simulink model "test_mdl1"  (R2023a)
settings: Solver=VariableStepAuto  StartTime=0.0  StopTime=10.0  RelTol=1e-3
(part 5 of 8)

== system test_mdl1/VehicleCAN/GWM/Power_Liftgate_Stat_FD1 ==
  DrLckCnt_No_ActlTgate : Constant  Value=0
  DrTGate_D_Rq : Constant  Value=0
  DrTgateChime2_D_Rq : Constant  Value=0
  Power_Liftgate_Mode_Stt : Constant  Value=0
  PwLftgtIntSw_B_Stat : Constant  Value=0
  bus_creator : BusCreator  Inputs=5
  out_port : Outport
  wires:
  bus_creator/1 -> out_port/1  "test_mdl1"
  DrLckCnt_No_ActlTgate/1 -> bus_creator/1  "DrLckCnt_No_ActlTgate"
  DrTGate_D_Rq/1 -> bus_creator/2  "DrTGate_D_Rq"
  DrTgateChime2_D_Rq/1 -> bus_creator/3  "DrTgateChime2_D_Rq"
  Power_Liftgate_Mode_Stt/1 -> bus_creator/4  "Power_Liftgate_Mode_Stt"
  PwLftgtIntSw_B_Stat/1 -> bus_creator/5  "PwLftgtIntSw_B_Stat"

== system test_mdl1/VehicleCAN/GWM/RCMSerialNumber_FD1 ==
  RCMSerialNoByte{1..8} (8 alike) : Constant  Value=0
  bus_creator : BusCreator  Inputs=8
  out_port : Outport
  wires:
  bus_creator/1 -> out_port/1  "test_mdl1"
  RCMSerialNoByte1/1 -> bus_creator/1  "RCMSerialNoByte1"
  RCMSerialNoByte2/1 -> bus_creator/2  "RCMSerialNoByte2"
  RCMSerialNoByte3/1 -> bus_creator/3  "RCMSerialNoByte3"
  RCMSerialNoByte4/1 -> bus_creator/4  "RCMSerialNoByte4"
  RCMSerialNoByte5/1 -> bus_creator/5  "RCMSerialNoByte5"
  RCMSerialNoByte6/1 -> bus_creator/6  "RCMSerialNoByte6"
  RCMSerialNoByte7/1 -> bus_creator/7  "RCMSerialNoByte7"
  RCMSerialNoByte8/1 -> bus_creator/8  "RCMSerialNoByte8"

== system test_mdl1/VehicleCAN/GWM/RCMStatusMessage2_FD1 ==
  EDRTriggerEvntSync : Constant  Value=0
  FirstRowBuckleDriver : Constant  Value=0
  FirstRowBuckleMid : Constant  Value=0
  FirstRowBucklePsngr : Constant  Value=0
  PassRstrnInd_Req : Constant  Value=0
  PsngrFrntDetct_D_Actl : Constant  Value=0
  RILReq : Constant  Value=0
  RstrnImpactEvntStatus : Constant  Value=0
  SecondRowBuckleDriver : Constant  Value=0
  SecondRowBuckleMid : Constant  Value=0
  SecondRowBucklePsngr : Constant  Value=0
  bus_creator : BusCreator  Inputs=11
  out_port : Outport
  wires:
  bus_creator/1 -> out_port/1  "test_mdl1"
  EDRTriggerEvntSync/1 -> bus_creator/1  "EDRTriggerEvntSync"
  FirstRowBuckleDriver/1 -> bus_creator/2  "FirstRowBuckleDriver"
  FirstRowBuckleMid/1 -> bus_creator/3  "FirstRowBuckleMid"
  FirstRowBucklePsngr/1 -> bus_creator/4  "FirstRowBucklePsngr"
  PassRstrnInd_Req/1 -> bus_creator/5  "PassRstrnInd_Req"
  PsngrFrntDetct_D_Actl/1 -> bus_creator/6  "PsngrFrntDetct_D_Actl"
  RILReq/1 -> bus_creator/7  "RILReq"
  RstrnImpactEvntStatus/1 -> bus_creator/8  "RstrnImpactEvntStatus"
  SecondRowBuckleDriver/1 -> bus_creator/9  "SecondRowBuckleDriver"
  SecondRowBuckleMid/1 -> bus_creator/10  "SecondRowBuckleMid"
  SecondRowBucklePsngr/1 -> bus_creator/11  "SecondRowBucklePsngr"

== system test_mdl1/VehicleCAN/GWM/SmartChargingData_ECG_1 ==
  ScLocDelete_B_RqCld : Constant  Value=0
  ScLocId_No_RqCld : Constant  Value=0
  ScLocLattDeg_An_RqCld : Constant  Value=0
  ScLocLattFrct_An_RqCld : Constant  Value=0
  ScLocLattPostv_B_RqCld : Constant  Value=0
  ScLocLongDeg_An_RqCld : Constant  Value=0
  ScLocLongFrct_An_RqCld : Constant  Value=0
  ScLocLongPostv_B_RqCld : Constant  Value=0
  bus_creator : BusCreator  Inputs=8
  out_port : Outport
  wires:
  bus_creator/1 -> out_port/1  "test_mdl1"
  ScLocDelete_B_RqCld/1 -> bus_creator/1  "ScLocDelete_B_RqCld"
  ScLocId_No_RqCld/1 -> bus_creator/2  "ScLocId_No_RqCld"
  ScLocLattDeg_An_RqCld/1 -> bus_creator/3  "ScLocLattDeg_An_RqCld"
  ScLocLattFrct_An_RqCld/1 -> bus_creator/4  "ScLocLattFrct_An_RqCld"
  ScLocLattPostv_B_RqCld/1 -> bus_creator/5  "ScLocLattPostv_B_RqCld"
  ScLocLongDeg_An_RqCld/1 -> bus_creator/6  "ScLocLongDeg_An_RqCld"
  ScLocLongFrct_An_RqCld/1 -> bus_creator/7  "ScLocLongFrct_An_RqCld"
  ScLocLongPostv_B_RqCld/1 -> bus_creator/8  "ScLocLongPostv_B_RqCld"

== system test_mdl1/VehicleCAN/GWM/SmartChargingData_ECG_2 ==
  ScChrgDurSet_D_RqCld : Constant  Value=0
  ScChrgDur_T_RqCld : Constant  Value=0
  ScChrgPrfl_No_RqCld : Constant  Value=0
  ScChrgToPc_Pc_RqCld : Constant  Value=0
  ScDayOfWeekId_D_RqCld : Constant  Value=0
  ScLocRdius_L_RqCld : Constant  Value=0
  ScLocSetId_No_RqCld : Constant  Value=0
  bus_creator : BusCreator  Inputs=7
  out_port : Outport
  wires:
  bus_creator/1 -> out_port/1  "test_mdl1"
  ScChrgDurSet_D_RqCld/1 -> bus_creator/1  "ScChrgDurSet_D_RqCld"
  ScChrgDur_T_RqCld/1 -> bus_creator/2  "ScChrgDur_T_RqCld"
  ScChrgPrfl_No_RqCld/1 -> bus_creator/3  "ScChrgPrfl_No_RqCld"
  ScChrgToPc_Pc_RqCld/1 -> bus_creator/4  "ScChrgToPc_Pc_RqCld"
  ScDayOfWeekId_D_RqCld/1 -> bus_creator/5  "ScDayOfWeekId_D_RqCld"
  ScLocRdius_L_RqCld/1 -> bus_creator/6  "ScLocRdius_L_RqCld"
  ScLocSetId_No_RqCld/1 -> bus_creator/7  "ScLocSetId_No_RqCld"

== system test_mdl1/VehicleCAN/GWM/SmartChargingData_ECG_3 ==
  AirAmb_Te_ActlCld : Constant  Value=0
  ChrgToPcEdit_Pc_RqCld : Constant  Value=0
  GoTEditHr_T_RqCld : Constant  Value=0
  GoTEditMnte_T_RqCld : Constant  Value=0
  PrcondEdit_D_RqCld : Constant  Value=0
  ScChrgrPwMax_Pw_RqCld : Constant  Value=0
  ScEnbl_D_RqCld : Constant  Value=0
  ScFreshDataEnbl_B_Rq : Constant  Value=0
  ScLocPwId_No_RqCld : Constant  Value=0
  ScMnSoc_Pc_RqCld : Constant  Value=0
  bus_creator : BusCreator  Inputs=10
  out_port : Outport
  wires:
  bus_creator/1 -> out_port/1  "test_mdl1"
  AirAmb_Te_ActlCld/1 -> bus_creator/1  "AirAmb_Te_ActlCld"
  ChrgToPcEdit_Pc_RqCld/1 -> bus_creator/2  "ChrgToPcEdit_Pc_RqCld"
  GoTEditHr_T_RqCld/1 -> bus_creator/3  "GoTEditHr_T_RqCld"
  GoTEditMnte_T_RqCld/1 -> bus_creator/4  "GoTEditMnte_T_RqCld"
  PrcondEdit_D_RqCld/1 -> bus_creator/5  "PrcondEdit_D_RqCld"
  ScChrgrPwMax_Pw_RqCld/1 -> bus_creator/6  "ScChrgrPwMax_Pw_RqCld"
  ScEnbl_D_RqCld/1 -> bus_creator/7  "ScEnbl_D_RqCld"
  ScFreshDataEnbl_B_Rq/1 -> bus_creator/8  "ScFreshDataEnbl_B_Rq"
  ScLocPwId_No_RqCld/1 -> bus_creator/9  "ScLocPwId_No_RqCld"
  ScMnSoc_Pc_RqCld/1 -> bus_creator/10  "ScMnSoc_Pc_RqCld"

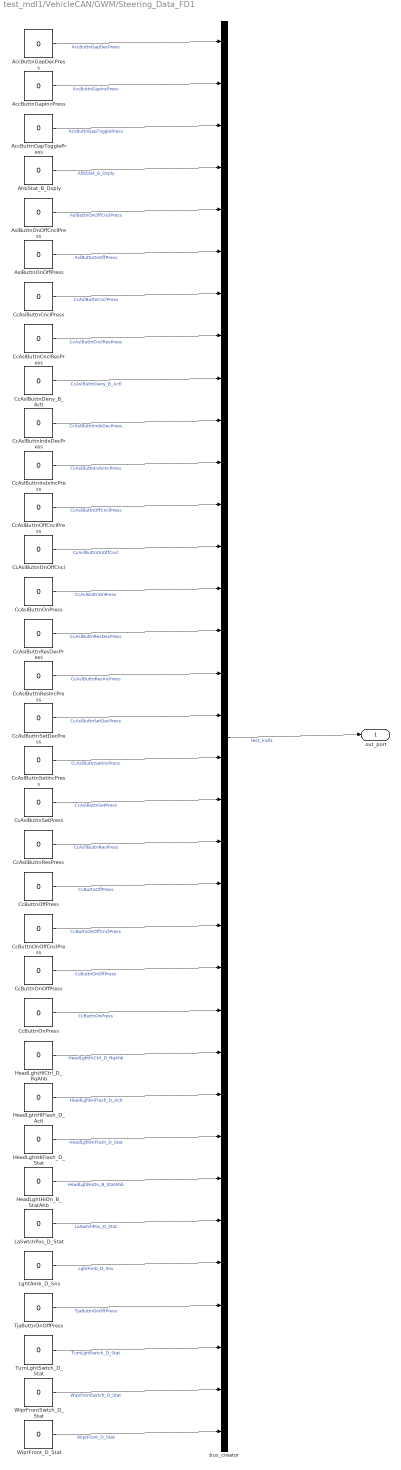
== system test_mdl1/VehicleCAN/GWM/Steering_Data_FD1 ==
  AccButtnGapDecPress : Constant  Value=0
  AccButtnGapIncPress : Constant  Value=0
  AccButtnGapTogglePress : Constant  Value=0
  AhbStat_B_Dsply : Constant  Value=0
  AslButtnOnOffCnclPress : Constant  Value=0
  AslButtnOnOffPress : Constant  Value=0
  CcAslButtnCnclPress : Constant  Value=0
  CcAslButtnCnclResPress : Constant  Value=0
  CcAslButtnDeny_B_Actl : Constant  Value=0
  CcAslButtnIndxDecPress : Constant  Value=0
  CcAslButtnIndxIncPress : Constant  Value=0
  CcAslButtnOffCnclPress : Constant  Value=0
  CcAslButtnOnOffCncl : Constant  Value=0
  CcAslButtnOnPress : Constant  Value=0
  CcAslButtnResDecPress : Constant  Value=0
  CcAslButtnResIncPress : Constant  Value=0
  CcAslButtnSetDecPress : Constant  Value=0
  CcAslButtnSetIncPress : Constant  Value=0
  CcAslButtnSetPress : Constant  Value=0
  CcAsllButtnResPress : Constant  Value=0
  CcButtnOffPress : Constant  Value=0
  CcButtnOnOffCnclPress : Constant  Value=0
  CcButtnOnOffPress : Constant  Value=0
  CcButtnOnPress : Constant  Value=0
  HeadLghtHiCtrl_D_RqAhb : Constant  Value=0
  HeadLghtHiFlash_D_Actl : Constant  Value=0
  HeadLghtHiFlash_D_Stat : Constant  Value=0
  HeadLghtHiOn_B_StatAhb : Constant  Value=0
  LaSwtchPos_D_Stat : Constant  Value=0
  LghtAmb_D_Sns : Constant  Value=0
  TjaButtnOnOffPress : Constant  Value=0
  TurnLghtSwtch_D_Stat : Constant  Value=0
  WiprFrontSwtch_D_Stat : Constant  Value=0
  WiprFront_D_Stat : Constant  Value=0
  bus_creator : BusCreator  Inputs=34
  out_port : Outport
  wires:
  bus_creator/1 -> out_port/1  "test_mdl1"
  AccButtnGapDecPress/1 -> bus_creator/1  "AccButtnGapDecPress"
  AccButtnGapIncPress/1 -> bus_creator/2  "AccButtnGapIncPress"
  AccButtnGapTogglePress/1 -> bus_creator/3  "AccButtnGapTogglePress"
  AhbStat_B_Dsply/1 -> bus_creator/4  "AhbStat_B_Dsply"
  AslButtnOnOffCnclPress/1 -> bus_creator/5  "AslButtnOnOffCnclPress"
  AslButtnOnOffPress/1 -> bus_creator/6  "AslButtnOnOffPress"
  CcAslButtnCnclPress/1 -> bus_creator/7  "CcAslButtnCnclPress"
  CcAslButtnCnclResPress/1 -> bus_creator/8  "CcAslButtnCnclResPress"
  CcAslButtnDeny_B_Actl/1 -> bus_creator/9  "CcAslButtnDeny_B_Actl"
  CcAslButtnIndxDecPress/1 -> bus_creator/10  "CcAslButtnIndxDecPress"
  CcAslButtnIndxIncPress/1 -> bus_creator/11  "CcAslButtnIndxIncPress"
  CcAslButtnOffCnclPress/1 -> bus_creator/12  "CcAslButtnOffCnclPress"
  CcAslButtnOnOffCncl/1 -> bus_creator/13  "CcAslButtnOnOffCncl"
  CcAslButtnOnPress/1 -> bus_creator/14  "CcAslButtnOnPress"
  CcAslButtnResDecPress/1 -> bus_creator/15  "CcAslButtnResDecPress"
  CcAslButtnResIncPress/1 -> bus_creator/16  "CcAslButtnResIncPress"
  CcAslButtnSetDecPress/1 -> bus_creator/17  "CcAslButtnSetDecPress"
  CcAslButtnSetIncPress/1 -> bus_creator/18  "CcAslButtnSetIncPress"
  CcAslButtnSetPress/1 -> bus_creator/19  "CcAslButtnSetPress"
  CcAsllButtnResPress/1 -> bus_creator/20  "CcAsllButtnResPress"
  CcButtnOffPress/1 -> bus_creator/21  "CcButtnOffPress"
  CcButtnOnOffCnclPress/1 -> bus_creator/22  "CcButtnOnOffCnclPress"
  CcButtnOnOffPress/1 -> bus_creator/23  "CcButtnOnOffPress"
  CcButtnOnPress/1 -> bus_creator/24  "CcButtnOnPress"
  HeadLghtHiCtrl_D_RqAhb/1 -> bus_creator/25  "HeadLghtHiCtrl_D_RqAhb"
  HeadLghtHiFlash_D_Actl/1 -> bus_creator/26  "HeadLghtHiFlash_D_Actl"
  HeadLghtHiFlash_D_Stat/1 -> bus_creator/27  "HeadLghtHiFlash_D_Stat"
  HeadLghtHiOn_B_StatAhb/1 -> bus_creator/28  "HeadLghtHiOn_B_StatAhb"
  LaSwtchPos_D_Stat/1 -> bus_creator/29  "LaSwtchPos_D_Stat"
  LghtAmb_D_Sns/1 -> bus_creator/30  "LghtAmb_D_Sns"
  TjaButtnOnOffPress/1 -> bus_creator/31  "TjaButtnOnOffPress"
  TurnLghtSwtch_D_Stat/1 -> bus_creator/32  "TurnLghtSwtch_D_Stat"
  WiprFrontSwtch_D_Stat/1 -> bus_creator/33  "WiprFrontSwtch_D_Stat"
  WiprFront_D_Stat/1 -> bus_creator/34  "WiprFront_D_Stat"

== system test_mdl1/VehicleCAN/GWM/Steering_Wheel_Data2_FD1 ==
  SelDrvMdeDec_B_RqDrv : Constant  Value=0
  SelDrvMdeInc_B_RqDrv : Constant  Value=0
  SelDrvMdeSwtch_D_Stat4 : Constant  Value=0
  SteEffortInc_B_RqDrv : Constant  Value=0
  SteWhlSwtchBack_B_Stat : Constant  Value=0
  SteWhlSwtchDown_B_Stat : Constant  Value=0
  SteWhlSwtchHome_B_Stat : Constant  Value=0
  SteWhlSwtchHud_B_Stat : Constant  Value=0
  SteWhlSwtchInfo_B_Stat : Constant  Value=0
  SteWhlSwtchIod_B_Stat : Constant  Value=0
  SteWhlSwtchLeft_B_Stat : Constant  Value=0
  SteWhlSwtchMed_B_Stat : Constant  Value=0
  SteWhlSwtchMenu_B_Stat : Constant  Value=0
  SteWhlSwtchNav_B_Stat : Constant  Value=0
  SteWhlSwtchOk_B_Stat : Constant  Value=0
  SteWhlSwtchPhon_B_Stat : Constant  Value=0
  SteWhlSwtchRght_B_Stat : Constant  Value=0
  SteWhlSwtchSet_B_Stat : Constant  Value=0
  SteWhlSwtchUp_B_Stat : Constant  Value=0
  SteWhlSwtchView_B_Stat : Constant  Value=0
  SuspDampInc_B_RqDrv : Constant  Value=0
  bus_creator : BusCreator  Inputs=21
  out_port : Outport
  wires:
  bus_creator/1 -> out_port/1  "test_mdl1"
  SelDrvMdeDec_B_RqDrv/1 -> bus_creator/1  "SelDrvMdeDec_B_RqDrv"
  SelDrvMdeInc_B_RqDrv/1 -> bus_creator/2  "SelDrvMdeInc_B_RqDrv"
  SelDrvMdeSwtch_D_Stat4/1 -> bus_creator/3  "SelDrvMdeSwtch_D_Stat4"
  SteEffortInc_B_RqDrv/1 -> bus_creator/4  "SteEffortInc_B_RqDrv"
  SteWhlSwtchBack_B_Stat/1 -> bus_creator/5  "SteWhlSwtchBack_B_Stat"
  SteWhlSwtchDown_B_Stat/1 -> bus_creator/6  "SteWhlSwtchDown_B_Stat"
  SteWhlSwtchHome_B_Stat/1 -> bus_creator/7  "SteWhlSwtchHome_B_Stat"
  SteWhlSwtchHud_B_Stat/1 -> bus_creator/8  "SteWhlSwtchHud_B_Stat"
  SteWhlSwtchInfo_B_Stat/1 -> bus_creator/9  "SteWhlSwtchInfo_B_Stat"
  SteWhlSwtchIod_B_Stat/1 -> bus_creator/10  "SteWhlSwtchIod_B_Stat"
  SteWhlSwtchLeft_B_Stat/1 -> bus_creator/11  "SteWhlSwtchLeft_B_Stat"
  SteWhlSwtchMed_B_Stat/1 -> bus_creator/12  "SteWhlSwtchMed_B_Stat"
  SteWhlSwtchMenu_B_Stat/1 -> bus_creator/13  "SteWhlSwtchMenu_B_Stat"
  SteWhlSwtchNav_B_Stat/1 -> bus_creator/14  "SteWhlSwtchNav_B_Stat"
  SteWhlSwtchOk_B_Stat/1 -> bus_creator/15  "SteWhlSwtchOk_B_Stat"
  SteWhlSwtchPhon_B_Stat/1 -> bus_creator/16  "SteWhlSwtchPhon_B_Stat"
  SteWhlSwtchRght_B_Stat/1 -> bus_creator/17  "SteWhlSwtchRght_B_Stat"
  SteWhlSwtchSet_B_Stat/1 -> bus_creator/18  "SteWhlSwtchSet_B_Stat"
  SteWhlSwtchUp_B_Stat/1 -> bus_creator/19  "SteWhlSwtchUp_B_Stat"
  SteWhlSwtchView_B_Stat/1 -> bus_creator/20  "SteWhlSwtchView_B_Stat"
  SuspDampInc_B_RqDrv/1 -> bus_creator/21  "SuspDampInc_B_RqDrv"

== system test_mdl1/VehicleCAN/GWM/TCU_Send_Signals_FD1 ==
  EmgcyCallMute_D_Stat : Constant  Value=0
  OfbChrgSetSync_D_Rq : Constant  Value=0
  TelematicsSrvc_D_St : Constant  Value=0
  bus_creator : BusCreator  Inputs=3
  out_port : Outport
  wires:
  bus_creator/1 -> out_port/1  "test_mdl1"
  EmgcyCallMute_D_Stat/1 -> bus_creator/1  "EmgcyCallMute_D_Stat"
  OfbChrgSetSync_D_Rq/1 -> bus_creator/2  "OfbChrgSetSync_D_Rq"
  TelematicsSrvc_D_St/1 -> bus_creator/3  "TelematicsSrvc_D_St"

== system test_mdl1/VehicleCAN/GWM/TesterPhysicalReqVDM_FD1 ==
  TesterPhysicalReqVDM : Constant  Value=0
  bus_creator : BusCreator  Inputs=1
  out_port : Outport
  wires:
  bus_creator/1 -> out_port/1  "test_mdl1"
  TesterPhysicalReqVDM/1 -> bus_creator/1  "TesterPhysicalReqVDM"

== system test_mdl1/VehicleCAN/GWM/TesterPhysicalResGWM_FD1 ==
  TesterPhysicalResGWM_F1 : Constant  Value=0
  bus_creator : BusCreator  Inputs=1
  out_port : Outport
  wires:
  bus_creator/1 -> out_port/1  "test_mdl1"
  TesterPhysicalResGWM_F1/1 -> bus_creator/1  "TesterPhysicalResGWM_F1"

== system test_mdl1/VehicleCAN/GWM/Tire_Pressure_Data_FD1 ==
  Tire_Press_LF_Data : Constant  Value=0
  Tire_Press_LR_OLR_Data : Constant  Value=0
  Tire_Press_RF_Data : Constant  Value=0
  Tire_Press_RR_ORR_Data : Constant  Value=0
  bus_creator : BusCreator  Inputs=4
  out_port : Outport
  wires:
  bus_creator/1 -> out_port/1  "test_mdl1"
  Tire_Press_LF_Data/1 -> bus_creator/1  "Tire_Press_LF_Data"
  Tire_Press_LR_OLR_Data/1 -> bus_creator/2  "Tire_Press_LR_OLR_Data"
  Tire_Press_RF_Data/1 -> bus_creator/3  "Tire_Press_RF_Data"
  Tire_Press_RR_ORR_Data/1 -> bus_creator/4  "Tire_Press_RR_ORR_Data"

== system test_mdl1/VehicleCAN/GWM/TrailerAid_Data3_FD1 ==
  TrlrAidEnbl_D2_Rq : Constant  Value=0
  TrlrAidSetup_D2_Rq : Constant  Value=0
  TrlrAnOffstDir_D_Mem : Constant  Value=0
  TrlrAnOffst_An_Mem : Constant  Value=0
  TrlrAxleToBmpr_L_Actl : Constant  Value=0
  TrlrBallToBmpr_L_Actl : Constant  Value=0
  TrlrIdType_D_Stat : Constant  Value=0
  TrlrId_No_Actl : Constant  Value=0
  TrlrRvrseCancl_B_Rq : Constant  Value=0
  TrlrTrgtOffst_L_Actl : Constant  Value=0
  TrlrTrgtPtrnId_No_Mem : Constant  Value=0
  TrlrTrgtToBmpr_L_Actl : Constant  Value=0
  bus_creator : BusCreator  Inputs=12
  out_port : Outport
  wires:
  bus_creator/1 -> out_port/1  "test_mdl1"
  TrlrAidEnbl_D2_Rq/1 -> bus_creator/1  "TrlrAidEnbl_D2_Rq"
  TrlrAidSetup_D2_Rq/1 -> bus_creator/2  "TrlrAidSetup_D2_Rq"
  TrlrAnOffstDir_D_Mem/1 -> bus_creator/3  "TrlrAnOffstDir_D_Mem"
  TrlrAnOffst_An_Mem/1 -> bus_creator/4  "TrlrAnOffst_An_Mem"
  TrlrAxleToBmpr_L_Actl/1 -> bus_creator/5  "TrlrAxleToBmpr_L_Actl"
  TrlrBallToBmpr_L_Actl/1 -> bus_creator/6  "TrlrBallToBmpr_L_Actl"
  TrlrIdType_D_Stat/1 -> bus_creator/7  "TrlrIdType_D_Stat"
  TrlrId_No_Actl/1 -> bus_creator/8  "TrlrId_No_Actl"
  TrlrRvrseCancl_B_Rq/1 -> bus_creator/9  "TrlrRvrseCancl_B_Rq"
  TrlrTrgtOffst_L_Actl/1 -> bus_creator/10  "TrlrTrgtOffst_L_Actl"
  TrlrTrgtPtrnId_No_Mem/1 -> bus_creator/11  "TrlrTrgtPtrnId_No_Mem"
  TrlrTrgtToBmpr_L_Actl/1 -> bus_creator/12  "TrlrTrgtToBmpr_L_Actl"

== system test_mdl1/VehicleCAN/GWM/TrailerAid_Data_FD1 ==
  TrailCtlSwtch_B_Stat2 : Constant  Value=0
  TrlBrkInitOut_D_Rq : Constant  Value=0
  bus_creator : BusCreator  Inputs=2
  out_port : Outport
  wires:
  bus_creator/1 -> out_port/1  "test_mdl1"
  TrailCtlSwtch_B_Stat2/1 -> bus_creator/1  "TrailCtlSwtch_B_Stat2"
  TrlBrkInitOut_D_Rq/1 -> bus_creator/2  "TrlBrkInitOut_D_Rq"

== system test_mdl1/VehicleCAN/GWM/TrailerAid_Stat1_FD1 ==
  TrlrSnsId_No_Actl : Constant  Value=0
  bus_creator : BusCreator  Inputs=1
  out_port : Outport
  wires:
  bus_creator/1 -> out_port/1  "test_mdl1"
  TrlrSnsId_No_Actl/1 -> bus_creator/1  "TrlrSnsId_No_Actl"

== system test_mdl1/VehicleCAN/GWM/TrailerAid_Stat2_FD1 ==
  TrlrHitYaw_AnRate_Actl : Constant  Value=0
  TrlrHitchYaw_An_Actl : Constant  Value=0
  TrlrHitchYaw_D_Stat : Constant  Value=0
  TrlrYawWActl_D_Qf : Constant  Value=0
  TrlrYaw_W_Actl : Constant  Value=0
  bus_creator : BusCreator  Inputs=5
  out_port : Outport
  wires:
  bus_creator/1 -> out_port/1  "test_mdl1"
  TrlrHitYaw_AnRate_Actl/1 -> bus_creator/1  "TrlrHitYaw_AnRate_Actl"
  TrlrHitchYaw_An_Actl/1 -> bus_creator/2  "TrlrHitchYaw_An_Actl"
  TrlrHitchYaw_D_Stat/1 -> bus_creator/3  "TrlrHitchYaw_D_Stat"
  TrlrYawWActl_D_Qf/1 -> bus_creator/4  "TrlrYawWActl_D_Qf"
  TrlrYaw_W_Actl/1 -> bus_creator/5  "TrlrYaw_W_Actl"

== system test_mdl1/VehicleCAN/GWM/TrailerBrakeInfo_FD1 ==
  StopLamp_B_RqTrlrBrk : Constant  Value=0
  TrlBrkInitOut_D_Stat : Constant  Value=0
  TrlrBrkActCirct_B_Falt : Constant  Value=0
  TrlrBrkActCnnct_B_Actl : Constant  Value=0
  TrlrBrkCtl_B_Falt : Constant  Value=0
  TrlrBrkDcnnt_B_Actl : Constant  Value=0
  TrlrBrkDsply_B_Rq : Constant  Value=0
  TrlrBrkGain_No_Actl : Constant  Value=0
  TrlrBrkMde_D_Actl : Constant  Value=0
  TrlrBrkOut_No_Dsply : Constant  Value=0
  bus_creator : BusCreator  Inputs=10
  out_port : Outport
  wires:
  bus_creator/1 -> out_port/1  "test_mdl1"
  StopLamp_B_RqTrlrBrk/1 -> bus_creator/1  "StopLamp_B_RqTrlrBrk"
  TrlBrkInitOut_D_Stat/1 -> bus_creator/2  "TrlBrkInitOut_D_Stat"
  TrlrBrkActCirct_B_Falt/1 -> bus_creator/3  "TrlrBrkActCirct_B_Falt"
  TrlrBrkActCnnct_B_Actl/1 -> bus_creator/4  "TrlrBrkActCnnct_B_Actl"
  TrlrBrkCtl_B_Falt/1 -> bus_creator/5  "TrlrBrkCtl_B_Falt"
  TrlrBrkDcnnt_B_Actl/1 -> bus_creator/6  "TrlrBrkDcnnt_B_Actl"
  TrlrBrkDsply_B_Rq/1 -> bus_creator/7  "TrlrBrkDsply_B_Rq"
  TrlrBrkGain_No_Actl/1 -> bus_creator/8  "TrlrBrkGain_No_Actl"
  TrlrBrkMde_D_Actl/1 -> bus_creator/9  "TrlrBrkMde_D_Actl"
  TrlrBrkOut_No_Dsply/1 -> bus_creator/10  "TrlrBrkOut_No_Dsply"

== system test_mdl1/VehicleCAN/GWM/TrailerInfo_2_FD1 ==
  TrlrAidCtl_U_RqDrv : Constant  Value=0
  TrlrAidSwtch_D_RqDrv : Constant  Value=0
  bus_creator : BusCreator  Inputs=2
  out_port : Outport
  wires:
  bus_creator/1 -> out_port/1  "test_mdl1"
  TrlrAidCtl_U_RqDrv/1 -> bus_creator/1  "TrlrAidCtl_U_RqDrv"
  TrlrAidSwtch_D_RqDrv/1 -> bus_creator/2  "TrlrAidSwtch_D_RqDrv"

== system test_mdl1/VehicleCAN/GWM/TrailerInfo_FD1 ==
  ParkLampTrlrOut_B_Stat : Constant  Value=0
  StopLampTrlrOut_B_Stat : Constant  Value=0
  TrlrBattChrg_D_Stat : Constant  Value=0
  TrlrLampCnnct_B_Actl : Constant  Value=0
  TrlrLampCtl_D_Stat : Constant  Value=0
  TurnLampTrlrRl_B_Stat : Constant  Value=0
  TurnLampTrlrRr_B_Stat : Constant  Value=0
  bus_creator : BusCreator  Inputs=7
  out_port : Outport
  wires:
  bus_creator/1 -> out_port/1  "test_mdl1"
  ParkLampTrlrOut_B_Stat/1 -> bus_creator/1  "ParkLampTrlrOut_B_Stat"
  StopLampTrlrOut_B_Stat/1 -> bus_creator/2  "StopLampTrlrOut_B_Stat"
  TrlrBattChrg_D_Stat/1 -> bus_creator/3  "TrlrBattChrg_D_Stat"
  TrlrLampCnnct_B_Actl/1 -> bus_creator/4  "TrlrLampCnnct_B_Actl"
  TrlrLampCtl_D_Stat/1 -> bus_creator/5  "TrlrLampCtl_D_Stat"
  TurnLampTrlrRl_B_Stat/1 -> bus_creator/6  "TurnLampTrlrRl_B_Stat"
  TurnLampTrlrRr_B_Stat/1 -> bus_creator/7  "TurnLampTrlrRr_B_Stat"

== system test_mdl1/VehicleCAN/GWM/Voltage_Power_Data2_FD1 ==
  CoolFanDcdc_D_Rq : Constant  Value=0
  DcdcClntFlw_D_Rq : Constant  Value=0
  bus_creator : BusCreator  Inputs=2
  out_port : Outport
  wires:
  bus_creator/1 -> out_port/1  "test_mdl1"
  CoolFanDcdc_D_Rq/1 -> bus_creator/1  "CoolFanDcdc_D_Rq"
  DcdcClntFlw_D_Rq/1 -> bus_creator/2  "DcdcClntFlw_D_Rq"

== system test_mdl1/VehicleCAN/GWM/Yaw_Data_FD1 ==
  VehRolWActl_D_Qf : Constant  Value=0
  VehRol_W_Actl : Constant  Value=0
  VehRollYawW_No_Cs : Constant  Value=0
  VehRollYaw_No_Cnt : Constant  Value=0
  VehYawWActl_D_Qf : Constant  Value=0
  VehYaw_W_Actl : Constant  Value=0
  bus_creator : BusCreator  Inputs=6
  out_port : Outport
  wires:
  bus_creator/1 -> out_port/1  "test_mdl1"
  VehRolWActl_D_Qf/1 -> bus_creator/1  "VehRolWActl_D_Qf"
  VehRol_W_Actl/1 -> bus_creator/2  "VehRol_W_Actl"
  VehRollYawW_No_Cs/1 -> bus_creator/3  "VehRollYawW_No_Cs"
  VehRollYaw_No_Cnt/1 -> bus_creator/4  "VehRollYaw_No_Cnt"
  VehYawWActl_D_Qf/1 -> bus_creator/5  "VehYawWActl_D_Qf"
  VehYaw_W_Actl/1 -> bus_creator/6  "VehYaw_W_Actl"

== system test_mdl1/VehicleCAN/IPMA_ADAS/%sonality_CCM_Data ==
  %sIndexCcm_D_Actl : Constant  Value=0
  FeatConfigCcmActl : Constant  Value=0
  FeatNoCcmActl : Constant  Value=0
  bus_creator : BusCreator  Inputs=3
  out_port : Outport
  wires:
  bus_creator/1 -> out_port/1  "test_mdl1"
  FeatConfigCcmActl/1 -> bus_creator/1  "FeatConfigCcmActl"
  FeatNoCcmActl/1 -> bus_creator/2  "FeatNoCcmActl"
  %sIndexCcm_D_Actl/1 -> bus_creator/3  "%sIndexCcm_D_Actl"

== system test_mdl1/VehicleCAN/IPMA_ADAS/%sonality_IPMB_Data ==
  %sIndexIpmb_D_Actl : Constant  Value=0
  FeatConfigIpmbActl : Constant  Value=0
  FeatNoIpmbActl : Constant  Value=0
  bus_creator : BusCreator  Inputs=3
  out_port : Outport
  wires:
  bus_creator/1 -> out_port/1  "test_mdl1"
  FeatConfigIpmbActl/1 -> bus_creator/1  "FeatConfigIpmbActl"
  FeatNoIpmbActl/1 -> bus_creator/2  "FeatNoIpmbActl"
  %sIndexIpmb_D_Actl/1 -> bus_creator/3  "%sIndexIpmb_D_Actl"

== system test_mdl1/VehicleCAN/IPMA_ADAS/ACCDATA ==
  AccAutoResum_D_Rq : Constant  Value=0
  AccBrkDecel_B_Rq : Constant  Value=0
  AccBrkPrchg_B_Rq : Constant  Value=0
  AccBrkPrkEl_B_Rq : Constant  Value=0
  AccBrkPulse_B_Rq : Constant  Value=0
  AccBrkTot_A_Rq : Constant  Value=0
  AccCancl_B_Rq : Constant  Value=0
  AccDeny_B_Rq : Constant  Value=0
  AccPrpl_A_Pred : Constant  Value=0
  AccPrpl_A_Rq : Constant  Value=0
  AccResumEnbl_B_Rq : Constant  Value=0
  AccStopStat_B_Rq : Constant  Value=0
  AccVeh_V_Trg : Constant  Value=0
  CmbbDeny_B_Actl : Constant  Value=0
  CmbbEngTqMn_B_Rq : Constant  Value=0
  CmbbOvrrd_B_RqDrv : Constant  Value=0
  Cmbb_B_Enbl : Constant  Value=0
  bus_creator : BusCreator  Inputs=17
  out_port : Outport
  wires:
  bus_creator/1 -> out_port/1  "test_mdl1"
  AccAutoResum_D_Rq/1 -> bus_creator/1  "AccAutoResum_D_Rq"
  AccBrkDecel_B_Rq/1 -> bus_creator/2  "AccBrkDecel_B_Rq"
  AccBrkPrchg_B_Rq/1 -> bus_creator/3  "AccBrkPrchg_B_Rq"
  AccBrkPrkEl_B_Rq/1 -> bus_creator/4  "AccBrkPrkEl_B_Rq"
  AccBrkPulse_B_Rq/1 -> bus_creator/5  "AccBrkPulse_B_Rq"
  AccBrkTot_A_Rq/1 -> bus_creator/6  "AccBrkTot_A_Rq"
  AccCancl_B_Rq/1 -> bus_creator/7  "AccCancl_B_Rq"
  AccDeny_B_Rq/1 -> bus_creator/8  "AccDeny_B_Rq"
  AccPrpl_A_Pred/1 -> bus_creator/9  "AccPrpl_A_Pred"
  AccPrpl_A_Rq/1 -> bus_creator/10  "AccPrpl_A_Rq"
  AccResumEnbl_B_Rq/1 -> bus_creator/11  "AccResumEnbl_B_Rq"
  AccStopStat_B_Rq/1 -> bus_creator/12  "AccStopStat_B_Rq"
  AccVeh_V_Trg/1 -> bus_creator/13  "AccVeh_V_Trg"
  CmbbDeny_B_Actl/1 -> bus_creator/14  "CmbbDeny_B_Actl"
  CmbbEngTqMn_B_Rq/1 -> bus_creator/15  "CmbbEngTqMn_B_Rq"
  CmbbOvrrd_B_RqDrv/1 -> bus_creator/16  "CmbbOvrrd_B_RqDrv"
  Cmbb_B_Enbl/1 -> bus_creator/17  "Cmbb_B_Enbl"

== system test_mdl1/VehicleCAN/IPMA_ADAS/ACCDATA_2 ==
  CmbbBaSens_D_Rq : Constant  Value=0
  CmbbBrkDecel_A_Rq : Constant  Value=0
  CmbbBrkDecel_B_Rq : Constant  Value=0
  CmbbBrkDecel_No_Cnt : Constant  Value=0
  CmbbBrkDecel_No_Cs : Constant  Value=0
  CmbbBrkPrchg_D_Rq : Constant  Value=0
  HudBlk1_B_Rq : Constant  Value=0
  HudBlk2_B_Rq : Constant  Value=0
  HudBlk3_B_Rq : Constant  Value=0
  HudDsplyIntns_No_Actl : Constant  Value=0
  HudFlashRate_D_Actl : Constant  Value=0
  bus_creator : BusCreator  Inputs=11
  out_port : Outport
  wires:
  bus_creator/1 -> out_port/1  "test_mdl1"
  CmbbBaSens_D_Rq/1 -> bus_creator/1  "CmbbBaSens_D_Rq"
  CmbbBrkDecel_A_Rq/1 -> bus_creator/2  "CmbbBrkDecel_A_Rq"
  CmbbBrkDecel_B_Rq/1 -> bus_creator/3  "CmbbBrkDecel_B_Rq"
  CmbbBrkDecel_No_Cnt/1 -> bus_creator/4  "CmbbBrkDecel_No_Cnt"
  CmbbBrkDecel_No_Cs/1 -> bus_creator/5  "CmbbBrkDecel_No_Cs"
  CmbbBrkPrchg_D_Rq/1 -> bus_creator/6  "CmbbBrkPrchg_D_Rq"
  HudBlk1_B_Rq/1 -> bus_creator/7  "HudBlk1_B_Rq"
  HudBlk2_B_Rq/1 -> bus_creator/8  "HudBlk2_B_Rq"
  HudBlk3_B_Rq/1 -> bus_creator/9  "HudBlk3_B_Rq"
  HudDsplyIntns_No_Actl/1 -> bus_creator/10  "HudDsplyIntns_No_Actl"
  HudFlashRate_D_Actl/1 -> bus_creator/11  "HudFlashRate_D_Actl"

== system test_mdl1/VehicleCAN/IPMA_ADAS/ACCDATA_3 ==
  AccFllwMde_B_Dsply : Constant  Value=0
  AccMemEnbl_B_RqDrv : Constant  Value=0
  AccMsgTxt_D2_Rq : Constant  Value=0
  AccStopMde_B_Dsply : Constant  Value=0
  AccStopRes_B_Dsply : Constant  Value=0
  AccStopStat_D_Dsply : Constant  Value=0
  AccTGap_B_Dsply : Constant  Value=0
  AccTGap_D_Dsply : Constant  Value=0
  AccTrgDist2_D_Dsply : Constant  Value=0
  AccWarn_D_Dsply : Constant  Value=0
  CadsAlignIncplt_B_Actl : Constant  Value=0
  CadsRadrBlck_B_Actl : Constant  Value=0
  CmbbPostEvnt_B_Dsply : Constant  Value=0
  FcwAudioWarn_B_Rq : Constant  Value=0
  FcwDeny_B_Dsply : Constant  Value=0
  FcwMemSens_D_Actl : Constant  Value=0
  FcwMemStat_B_Actl : Constant  Value=0
  FcwMsgTxt_D_Rq : Constant  Value=0
  FcwVisblWarn_B_Rq : Constant  Value=0
  FdaMem_B_Stat : Constant  Value=0
  HaDsply_No_Cnt : Constant  Value=0
  HaDsply_No_Cs : Constant  Value=0
  IaccLamp_D_Rq : Constant  Value=0
  TjaMsgTxt_D_Dsply : Constant  Value=0
  TjaWarn_D_Rq : Constant  Value=0
  Tja_D_Stat : Constant  Value=0
  bus_creator : BusCreator  Inputs=26
  out_port : Outport
  wires:
  bus_creator/1 -> out_port/1  "test_mdl1"
  AccFllwMde_B_Dsply/1 -> bus_creator/1  "AccFllwMde_B_Dsply"
  AccMemEnbl_B_RqDrv/1 -> bus_creator/2  "AccMemEnbl_B_RqDrv"
  AccMsgTxt_D2_Rq/1 -> bus_creator/3  "AccMsgTxt_D2_Rq"
  AccStopMde_B_Dsply/1 -> bus_creator/4  "AccStopMde_B_Dsply"
  AccStopRes_B_Dsply/1 -> bus_creator/5  "AccStopRes_B_Dsply"
  AccStopStat_D_Dsply/1 -> bus_creator/6  "AccStopStat_D_Dsply"
  AccTGap_B_Dsply/1 -> bus_creator/7  "AccTGap_B_Dsply"
  AccTGap_D_Dsply/1 -> bus_creator/8  "AccTGap_D_Dsply"
  AccTrgDist2_D_Dsply/1 -> bus_creator/9  "AccTrgDist2_D_Dsply"
  AccWarn_D_Dsply/1 -> bus_creator/10  "AccWarn_D_Dsply"
  CadsAlignIncplt_B_Actl/1 -> bus_creator/11  "CadsAlignIncplt_B_Actl"
  CadsRadrBlck_B_Actl/1 -> bus_creator/12  "CadsRadrBlck_B_Actl"
  CmbbPostEvnt_B_Dsply/1 -> bus_creator/13  "CmbbPostEvnt_B_Dsply"
  FcwAudioWarn_B_Rq/1 -> bus_creator/14  "FcwAudioWarn_B_Rq"
  FcwDeny_B_Dsply/1 -> bus_creator/15  "FcwDeny_B_Dsply"
  FcwMemSens_D_Actl/1 -> bus_creator/16  "FcwMemSens_D_Actl"
  FcwMemStat_B_Actl/1 -> bus_creator/17  "FcwMemStat_B_Actl"
  FcwMsgTxt_D_Rq/1 -> bus_creator/18  "FcwMsgTxt_D_Rq"
  FcwVisblWarn_B_Rq/1 -> bus_creator/19  "FcwVisblWarn_B_Rq"
  FdaMem_B_Stat/1 -> bus_creator/20  "FdaMem_B_Stat"
  HaDsply_No_Cnt/1 -> bus_creator/21  "HaDsply_No_Cnt"
  HaDsply_No_Cs/1 -> bus_creator/22  "HaDsply_No_Cs"
  IaccLamp_D_Rq/1 -> bus_creator/23  "IaccLamp_D_Rq"
  TjaMsgTxt_D_Dsply/1 -> bus_creator/24  "TjaMsgTxt_D_Dsply"
  TjaWarn_D_Rq/1 -> bus_creator/25  "TjaWarn_D_Rq"
  Tja_D_Stat/1 -> bus_creator/26  "Tja_D_Stat"

== system test_mdl1/VehicleCAN/IPMA_ADAS/AutoDriveBeam_Data1 ==
  AdbBrdr1CritLeft_T_Stat : Constant  Value=0
  AdbBrdr1CritRigh_T_Stat : Constant  Value=0
  AdbBrdr1DistLeft_D_Stat : Constant  Value=0
  AdbBrdr1DistRigh_D_Stat : Constant  Value=0
  AdbBrdr1Left_An_Rq : Constant  Value=0
  AdbBrdr1Low_An_Rq : Constant  Value=0
  AdbBrdr1Right_An_Rq : Constant  Value=0
  AdbBrdr1Up_An_Rq : Constant  Value=0
  AdbIntns1_D_Rq : Constant  Value=0
  AdbMde1_D_Rq : Constant  Value=0
  bus_creator : BusCreator  Inputs=10
  out_port : Outport
  wires:
  bus_creator/1 -> out_port/1  "test_mdl1"
  AdbBrdr1CritLeft_T_Stat/1 -> bus_creator/1  "AdbBrdr1CritLeft_T_Stat"
  AdbBrdr1CritRigh_T_Stat/1 -> bus_creator/2  "AdbBrdr1CritRigh_T_Stat"
  AdbBrdr1DistLeft_D_Stat/1 -> bus_creator/3  "AdbBrdr1DistLeft_D_Stat"
  AdbBrdr1DistRigh_D_Stat/1 -> bus_creator/4  "AdbBrdr1DistRigh_D_Stat"
  AdbBrdr1Left_An_Rq/1 -> bus_creator/5  "AdbBrdr1Left_An_Rq"
  AdbBrdr1Low_An_Rq/1 -> bus_creator/6  "AdbBrdr1Low_An_Rq"
  AdbBrdr1Right_An_Rq/1 -> bus_creator/7  "AdbBrdr1Right_An_Rq"
  AdbBrdr1Up_An_Rq/1 -> bus_creator/8  "AdbBrdr1Up_An_Rq"
  AdbIntns1_D_Rq/1 -> bus_creator/9  "AdbIntns1_D_Rq"
  AdbMde1_D_Rq/1 -> bus_creator/10  "AdbMde1_D_Rq"

== system test_mdl1/VehicleCAN/IPMA_ADAS/AutoDriveBeam_Data2 ==
  AdbBrdr2CritLeft_T_Stat : Constant  Value=0
  AdbBrdr2CritRigh_T_Stat : Constant  Value=0
  AdbBrdr2DistLeft_D_Stat : Constant  Value=0
  AdbBrdr2DistRigh_D_Stat : Constant  Value=0
  AdbBrdr2Left_An_Rq : Constant  Value=0
  AdbBrdr2Low_An_Rq : Constant  Value=0
  AdbBrdr2Right_An_Rq : Constant  Value=0
  AdbBrdr2Up_An_Rq : Constant  Value=0
  AdbIntns2_D_Rq : Constant  Value=0
  AdbMde2_D_Rq : Constant  Value=0
  bus_creator : BusCreator  Inputs=10
  out_port : Outport
  wires:
  bus_creator/1 -> out_port/1  "test_mdl1"
  AdbBrdr2CritLeft_T_Stat/1 -> bus_creator/1  "AdbBrdr2CritLeft_T_Stat"
  AdbBrdr2CritRigh_T_Stat/1 -> bus_creator/2  "AdbBrdr2CritRigh_T_Stat"
  AdbBrdr2DistLeft_D_Stat/1 -> bus_creator/3  "AdbBrdr2DistLeft_D_Stat"
  AdbBrdr2DistRigh_D_Stat/1 -> bus_creator/4  "AdbBrdr2DistRigh_D_Stat"
  AdbBrdr2Left_An_Rq/1 -> bus_creator/5  "AdbBrdr2Left_An_Rq"
  AdbBrdr2Low_An_Rq/1 -> bus_creator/6  "AdbBrdr2Low_An_Rq"
  AdbBrdr2Right_An_Rq/1 -> bus_creator/7  "AdbBrdr2Right_An_Rq"
  AdbBrdr2Up_An_Rq/1 -> bus_creator/8  "AdbBrdr2Up_An_Rq"
  AdbIntns2_D_Rq/1 -> bus_creator/9  "AdbIntns2_D_Rq"
  AdbMde2_D_Rq/1 -> bus_creator/10  "AdbMde2_D_Rq"

== system test_mdl1/VehicleCAN/IPMA_ADAS/AutoDriveBeam_Data3 ==
  AdbBrdr3CritLeft_T_Stat : Constant  Value=0
  AdbBrdr3CritRigh_T_Stat : Constant  Value=0
  AdbBrdr3DistLeft_D_Stat : Constant  Value=0
  AdbBrdr3DistRigh_D_Stat : Constant  Value=0
  AdbBrdr3Left_An_Rq : Constant  Value=0
  AdbBrdr3Low_An_Rq : Constant  Value=0
  AdbBrdr3Right_An_Rq : Constant  Value=0
  AdbBrdr3Up_An_Rq : Constant  Value=0
  AdbIntns3_D_Rq : Constant  Value=0
  AdbMde3_D_Rq : Constant  Value=0
  bus_creator : BusCreator  Inputs=10
  out_port : Outport
  wires:
  bus_creator/1 -> out_port/1  "test_mdl1"
  AdbBrdr3CritLeft_T_Stat/1 -> bus_creator/1  "AdbBrdr3CritLeft_T_Stat"
  AdbBrdr3CritRigh_T_Stat/1 -> bus_creator/2  "AdbBrdr3CritRigh_T_Stat"
  AdbBrdr3DistLeft_D_Stat/1 -> bus_creator/3  "AdbBrdr3DistLeft_D_Stat"
  AdbBrdr3DistRigh_D_Stat/1 -> bus_creator/4  "AdbBrdr3DistRigh_D_Stat"
  AdbBrdr3Left_An_Rq/1 -> bus_creator/5  "AdbBrdr3Left_An_Rq"
  AdbBrdr3Low_An_Rq/1 -> bus_creator/6  "AdbBrdr3Low_An_Rq"
  AdbBrdr3Right_An_Rq/1 -> bus_creator/7  "AdbBrdr3Right_An_Rq"
  AdbBrdr3Up_An_Rq/1 -> bus_creator/8  "AdbBrdr3Up_An_Rq"
  AdbIntns3_D_Rq/1 -> bus_creator/9  "AdbIntns3_D_Rq"
  AdbMde3_D_Rq/1 -> bus_creator/10  "AdbMde3_D_Rq"

== system test_mdl1/VehicleCAN/IPMA_ADAS/Bndry_Alert_L_Data ==
  BalrChimeLeft_D_Rq : Constant  Value=0
  BalrLckLeft_B_Stat : Constant  Value=0
  BalrLeft_D_Stat : Constant  Value=0
  BalrMdeLeft_D_Stat : Constant  Value=0
  BalrMdeSelLeft_B_Stat : Constant  Value=0
  BalrSnsLeft_D_Falt : Constant  Value=0
  BalrWndwLeft_B_Stat : Constant  Value=0
  CamraRearOn_B_RqBalrl : Constant  Value=0
  DrLckActv_B_RqBalrl : Constant  Value=0
  DrLckCnt_No_ActlBalrl : Constant  Value=0
  WndwDrvRear_D_RqBalrl : Constant  Value=0
  WndwDrv_D_RqBalrl : Constant  Value=0
  WndwPsngrRear_D_RqBalrl : Constant  Value=0
  WndwPsngr_D_RqBalrl : Constant  Value=0
  bus_creator : BusCreator  Inputs=14
  out_port : Outport
  wires:
  bus_creator/1 -> out_port/1  "test_mdl1"
  BalrChimeLeft_D_Rq/1 -> bus_creator/1  "BalrChimeLeft_D_Rq"
  BalrLckLeft_B_Stat/1 -> bus_creator/2  "BalrLckLeft_B_Stat"
  BalrLeft_D_Stat/1 -> bus_creator/3  "BalrLeft_D_Stat"
  BalrMdeLeft_D_Stat/1 -> bus_creator/4  "BalrMdeLeft_D_Stat"
  BalrMdeSelLeft_B_Stat/1 -> bus_creator/5  "BalrMdeSelLeft_B_Stat"
  BalrSnsLeft_D_Falt/1 -> bus_creator/6  "BalrSnsLeft_D_Falt"
  BalrWndwLeft_B_Stat/1 -> bus_creator/7  "BalrWndwLeft_B_Stat"
  CamraRearOn_B_RqBalrl/1 -> bus_creator/8  "CamraRearOn_B_RqBalrl"
  DrLckActv_B_RqBalrl/1 -> bus_creator/9  "DrLckActv_B_RqBalrl"
  DrLckCnt_No_ActlBalrl/1 -> bus_creator/10  "DrLckCnt_No_ActlBalrl"
  WndwDrvRear_D_RqBalrl/1 -> bus_creator/11  "WndwDrvRear_D_RqBalrl"
  WndwDrv_D_RqBalrl/1 -> bus_creator/12  "WndwDrv_D_RqBalrl"
  WndwPsngrRear_D_RqBalrl/1 -> bus_creator/13  "WndwPsngrRear_D_RqBalrl"
  WndwPsngr_D_RqBalrl/1 -> bus_creator/14  "WndwPsngr_D_RqBalrl"

== system test_mdl1/VehicleCAN/IPMA_ADAS/Bndry_Alert_R_Data ==
  BalrChimeRight_D_Rq : Constant  Value=0
  BalrLckRight_B_Stat : Constant  Value=0
  BalrMdeRight_D_Stat : Constant  Value=0
  BalrMdeSelRight_B_Stat : Constant  Value=0
  BalrRight_D_Stat : Constant  Value=0
  BalrSnsRight_D_Falt : Constant  Value=0
  BalrWndwRight_B_Stat : Constant  Value=0
  CamraRearOn_B_RqBalrr : Constant  Value=0
  DrLckActv_B_RqBalrr : Constant  Value=0
  DrLckCnt_No_ActlBalrr : Constant  Value=0
  WndwDrvRear_D_RqBalrr : Constant  Value=0
  WndwDrv_D_RqBalrr : Constant  Value=0
  WndwPsngrRear_D_RqBalrr : Constant  Value=0
  WndwPsngr_D_RqBalrr : Constant  Value=0
  bus_creator : BusCreator  Inputs=14
  out_port : Outport
  wires:
  bus_creator/1 -> out_port/1  "test_mdl1"
  BalrChimeRight_D_Rq/1 -> bus_creator/1  "BalrChimeRight_D_Rq"
  BalrLckRight_B_Stat/1 -> bus_creator/2  "BalrLckRight_B_Stat"
  BalrMdeRight_D_Stat/1 -> bus_creator/3  "BalrMdeRight_D_Stat"
  BalrMdeSelRight_B_Stat/1 -> bus_creator/4  "BalrMdeSelRight_B_Stat"
  BalrRight_D_Stat/1 -> bus_creator/5  "BalrRight_D_Stat"
  BalrSnsRight_D_Falt/1 -> bus_creator/6  "BalrSnsRight_D_Falt"
  BalrWndwRight_B_Stat/1 -> bus_creator/7  "BalrWndwRight_B_Stat"
  CamraRearOn_B_RqBalrr/1 -> bus_creator/8  "CamraRearOn_B_RqBalrr"
  DrLckActv_B_RqBalrr/1 -> bus_creator/9  "DrLckActv_B_RqBalrr"
  DrLckCnt_No_ActlBalrr/1 -> bus_creator/10  "DrLckCnt_No_ActlBalrr"
  WndwDrvRear_D_RqBalrr/1 -> bus_creator/11  "WndwDrvRear_D_RqBalrr"
  WndwDrv_D_RqBalrr/1 -> bus_creator/12  "WndwDrv_D_RqBalrr"
  WndwPsngrRear_D_RqBalrr/1 -> bus_creator/13  "WndwPsngrRear_D_RqBalrr"
  WndwPsngr_D_RqBalrr/1 -> bus_creator/14  "WndwPsngr_D_RqBalrr"

== system test_mdl1/VehicleCAN/IPMA_ADAS/BoundaryAlert_Left_1 ==
  BalrLeft1CurntX_L_Actl : Constant  Value=0
  BalrLeft1CurntY_L_Actl : Constant  Value=0
  BalrLeft1Dsply_B_Stat : Constant  Value=0
  BalrLeft1Fast_B_Stat : Constant  Value=0
  BalrLeft1Prev1X_L_Actl : Constant  Value=0
  BalrLeft1Prev1Y_L_Actl : Constant  Value=0
  BalrLeft1Prev2X_L_Actl : Constant  Value=0
  BalrLeft1Prev2Y_L_Actl : Constant  Value=0
  BalrLeft1Prev3X_L_Actl : Constant  Value=0
  BalrLeft1Prev3Y_L_Actl : Constant  Value=0
  BalrLeft1Threat_D_Stat : Constant  Value=0
  bus_creator : BusCreator  Inputs=11
  out_port : Outport
  wires:
  bus_creator/1 -> out_port/1  "test_mdl1"
  BalrLeft1CurntX_L_Actl/1 -> bus_creator/1  "BalrLeft1CurntX_L_Actl"
  BalrLeft1CurntY_L_Actl/1 -> bus_creator/2  "BalrLeft1CurntY_L_Actl"
  BalrLeft1Dsply_B_Stat/1 -> bus_creator/3  "BalrLeft1Dsply_B_Stat"
  BalrLeft1Fast_B_Stat/1 -> bus_creator/4  "BalrLeft1Fast_B_Stat"
  BalrLeft1Prev1X_L_Actl/1 -> bus_creator/5  "BalrLeft1Prev1X_L_Actl"
  BalrLeft1Prev1Y_L_Actl/1 -> bus_creator/6  "BalrLeft1Prev1Y_L_Actl"
  BalrLeft1Prev2X_L_Actl/1 -> bus_creator/7  "BalrLeft1Prev2X_L_Actl"
  BalrLeft1Prev2Y_L_Actl/1 -> bus_creator/8  "BalrLeft1Prev2Y_L_Actl"
  BalrLeft1Prev3X_L_Actl/1 -> bus_creator/9  "BalrLeft1Prev3X_L_Actl"
  BalrLeft1Prev3Y_L_Actl/1 -> bus_creator/10  "BalrLeft1Prev3Y_L_Actl"
  BalrLeft1Threat_D_Stat/1 -> bus_creator/11  "BalrLeft1Threat_D_Stat"

== system test_mdl1/VehicleCAN/IPMA_ADAS/BoundaryAlert_Left_2 ==
  BalrLeft2CurntX_L_Actl : Constant  Value=0
  BalrLeft2CurntY_L_Actl : Constant  Value=0
  BalrLeft2Dsply_B_Stat : Constant  Value=0
  BalrLeft2Fast_B_Stat : Constant  Value=0
  BalrLeft2Prev1X_L_Actl : Constant  Value=0
  BalrLeft2Prev1Y_L_Actl : Constant  Value=0
  BalrLeft2Prev2X_L_Actl : Constant  Value=0
  BalrLeft2Prev2Y_L_Actl : Constant  Value=0
  BalrLeft2Prev3X_L_Actl : Constant  Value=0
  BalrLeft2Prev3Y_L_Actl : Constant  Value=0
  BalrLeft2Threat_D_Stat : Constant  Value=0
  bus_creator : BusCreator  Inputs=11
  out_port : Outport
  wires:
  bus_creator/1 -> out_port/1  "test_mdl1"
  BalrLeft2CurntX_L_Actl/1 -> bus_creator/1  "BalrLeft2CurntX_L_Actl"
  BalrLeft2CurntY_L_Actl/1 -> bus_creator/2  "BalrLeft2CurntY_L_Actl"
  BalrLeft2Dsply_B_Stat/1 -> bus_creator/3  "BalrLeft2Dsply_B_Stat"
  BalrLeft2Fast_B_Stat/1 -> bus_creator/4  "BalrLeft2Fast_B_Stat"
  BalrLeft2Prev1X_L_Actl/1 -> bus_creator/5  "BalrLeft2Prev1X_L_Actl"
  BalrLeft2Prev1Y_L_Actl/1 -> bus_creator/6  "BalrLeft2Prev1Y_L_Actl"
  BalrLeft2Prev2X_L_Actl/1 -> bus_creator/7  "BalrLeft2Prev2X_L_Actl"
  BalrLeft2Prev2Y_L_Actl/1 -> bus_creator/8  "BalrLeft2Prev2Y_L_Actl"
  BalrLeft2Prev3X_L_Actl/1 -> bus_creator/9  "BalrLeft2Prev3X_L_Actl"
  BalrLeft2Prev3Y_L_Actl/1 -> bus_creator/10  "BalrLeft2Prev3Y_L_Actl"
  BalrLeft2Threat_D_Stat/1 -> bus_creator/11  "BalrLeft2Threat_D_Stat"

== system test_mdl1/VehicleCAN/IPMA_ADAS/BoundaryAlert_Left_3 ==
  BalrLeft3CurntX_L_Actl : Constant  Value=0
  BalrLeft3CurntY_L_Actl : Constant  Value=0
  BalrLeft3Dsply_B_Stat : Constant  Value=0
  BalrLeft3Fast_B_Stat : Constant  Value=0
  BalrLeft3Prev1X_L_Actl : Constant  Value=0
  BalrLeft3Prev1Y_L_Actl : Constant  Value=0
  BalrLeft3Prev2X_L_Actl : Constant  Value=0
  BalrLeft3Prev2Y_L_Actl : Constant  Value=0
  BalrLeft3Prev3X_L_Actl : Constant  Value=0
  BalrLeft3Prev3Y_L_Actl : Constant  Value=0
  BalrLeft3Threat_D_Stat : Constant  Value=0
  bus_creator : BusCreator  Inputs=11
  out_port : Outport
  wires:
  bus_creator/1 -> out_port/1  "test_mdl1"
  BalrLeft3CurntX_L_Actl/1 -> bus_creator/1  "BalrLeft3CurntX_L_Actl"
  BalrLeft3CurntY_L_Actl/1 -> bus_creator/2  "BalrLeft3CurntY_L_Actl"
  BalrLeft3Dsply_B_Stat/1 -> bus_creator/3  "BalrLeft3Dsply_B_Stat"
  BalrLeft3Fast_B_Stat/1 -> bus_creator/4  "BalrLeft3Fast_B_Stat"
  BalrLeft3Prev1X_L_Actl/1 -> bus_creator/5  "BalrLeft3Prev1X_L_Actl"
  BalrLeft3Prev1Y_L_Actl/1 -> bus_creator/6  "BalrLeft3Prev1Y_L_Actl"
  BalrLeft3Prev2X_L_Actl/1 -> bus_creator/7  "BalrLeft3Prev2X_L_Actl"
  BalrLeft3Prev2Y_L_Actl/1 -> bus_creator/8  "BalrLeft3Prev2Y_L_Actl"
  BalrLeft3Prev3X_L_Actl/1 -> bus_creator/9  "BalrLeft3Prev3X_L_Actl"
  BalrLeft3Prev3Y_L_Actl/1 -> bus_creator/10  "BalrLeft3Prev3Y_L_Actl"
  BalrLeft3Threat_D_Stat/1 -> bus_creator/11  "BalrLeft3Threat_D_Stat"

== system test_mdl1/VehicleCAN/IPMA_ADAS/BoundaryAlert_Left_4 ==
  BalrLeft4CurntX_L_Actl : Constant  Value=0
  BalrLeft4CurntY_L_Actl : Constant  Value=0
  BalrLeft4Dsply_B_Stat : Constant  Value=0
  BalrLeft4Fast_B_Stat : Constant  Value=0
  BalrLeft4Prev1X_L_Actl : Constant  Value=0
  BalrLeft4Prev1Y_L_Actl : Constant  Value=0
  BalrLeft4Prev2X_L_Actl : Constant  Value=0
  BalrLeft4Prev2Y_L_Actl : Constant  Value=0
  BalrLeft4Prev3X_L_Actl : Constant  Value=0
  BalrLeft4Prev3Y_L_Actl : Constant  Value=0
  BalrLeft4Threat_D_Stat : Constant  Value=0
  bus_creator : BusCreator  Inputs=11
  out_port : Outport
  wires:
  bus_creator/1 -> out_port/1  "test_mdl1"
  BalrLeft4CurntX_L_Actl/1 -> bus_creator/1  "BalrLeft4CurntX_L_Actl"
  BalrLeft4CurntY_L_Actl/1 -> bus_creator/2  "BalrLeft4CurntY_L_Actl"
  BalrLeft4Dsply_B_Stat/1 -> bus_creator/3  "BalrLeft4Dsply_B_Stat"
  BalrLeft4Fast_B_Stat/1 -> bus_creator/4  "BalrLeft4Fast_B_Stat"
  BalrLeft4Prev1X_L_Actl/1 -> bus_creator/5  "BalrLeft4Prev1X_L_Actl"
  BalrLeft4Prev1Y_L_Actl/1 -> bus_creator/6  "BalrLeft4Prev1Y_L_Actl"
  BalrLeft4Prev2X_L_Actl/1 -> bus_creator/7  "BalrLeft4Prev2X_L_Actl"
  BalrLeft4Prev2Y_L_Actl/1 -> bus_creator/8  "BalrLeft4Prev2Y_L_Actl"
  BalrLeft4Prev3X_L_Actl/1 -> bus_creator/9  "BalrLeft4Prev3X_L_Actl"
  BalrLeft4Prev3Y_L_Actl/1 -> bus_creator/10  "BalrLeft4Prev3Y_L_Actl"
  BalrLeft4Threat_D_Stat/1 -> bus_creator/11  "BalrLeft4Threat_D_Stat"

== system test_mdl1/VehicleCAN/IPMA_ADAS/BoundaryAlert_Right_1 ==
  BalrRight1CurntX_L_Actl : Constant  Value=0
  BalrRight1CurntY_L_Actl : Constant  Value=0
  BalrRight1Dsply_B_Stat : Constant  Value=0
  BalrRight1Fast_B_Stat : Constant  Value=0
  BalrRight1Prev1X_L_Actl : Constant  Value=0
  BalrRight1Prev1Y_L_Actl : Constant  Value=0
  BalrRight1Prev2X_L_Actl : Constant  Value=0
  BalrRight1Prev2Y_L_Actl : Constant  Value=0
  BalrRight1Prev3X_L_Actl : Constant  Value=0
  BalrRight1Prev3Y_L_Actl : Constant  Value=0
  BalrRight1Threat_D_Stat : Constant  Value=0
  bus_creator : BusCreator  Inputs=11
  out_port : Outport
  wires:
  bus_creator/1 -> out_port/1  "test_mdl1"
  BalrRight1CurntX_L_Actl/1 -> bus_creator/1  "BalrRight1CurntX_L_Actl"
  BalrRight1CurntY_L_Actl/1 -> bus_creator/2  "BalrRight1CurntY_L_Actl"
  BalrRight1Dsply_B_Stat/1 -> bus_creator/3  "BalrRight1Dsply_B_Stat"
  BalrRight1Fast_B_Stat/1 -> bus_creator/4  "BalrRight1Fast_B_Stat"
  BalrRight1Prev1X_L_Actl/1 -> bus_creator/5  "BalrRight1Prev1X_L_Actl"
  BalrRight1Prev1Y_L_Actl/1 -> bus_creator/6  "BalrRight1Prev1Y_L_Actl"
  BalrRight1Prev2X_L_Actl/1 -> bus_creator/7  "BalrRight1Prev2X_L_Actl"
  BalrRight1Prev2Y_L_Actl/1 -> bus_creator/8  "BalrRight1Prev2Y_L_Actl"
  BalrRight1Prev3X_L_Actl/1 -> bus_creator/9  "BalrRight1Prev3X_L_Actl"
  BalrRight1Prev3Y_L_Actl/1 -> bus_creator/10  "BalrRight1Prev3Y_L_Actl"
  BalrRight1Threat_D_Stat/1 -> bus_creator/11  "BalrRight1Threat_D_Stat"

== system test_mdl1/VehicleCAN/IPMA_ADAS/BoundaryAlert_Right_2 ==
  BalrRight2CurntX_L_Actl : Constant  Value=0
  BalrRight2CurntY_L_Actl : Constant  Value=0
  BalrRight2Dsply_B_Stat : Constant  Value=0
  BalrRight2Fast_B_Stat : Constant  Value=0
  BalrRight2Prev1X_L_Actl : Constant  Value=0
  BalrRight2Prev1Y_L_Actl : Constant  Value=0
  BalrRight2Prev2X_L_Actl : Constant  Value=0
  BalrRight2Prev2Y_L_Actl : Constant  Value=0
  BalrRight2Prev3X_L_Actl : Constant  Value=0
  BalrRight2Prev3Y_L_Actl : Constant  Value=0
  BalrRight2Threat_D_Stat : Constant  Value=0
  bus_creator : BusCreator  Inputs=11
  out_port : Outport
  wires:
  bus_creator/1 -> out_port/1  "test_mdl1"
  BalrRight2CurntX_L_Actl/1 -> bus_creator/1  "BalrRight2CurntX_L_Actl"
  BalrRight2CurntY_L_Actl/1 -> bus_creator/2  "BalrRight2CurntY_L_Actl"
  BalrRight2Dsply_B_Stat/1 -> bus_creator/3  "BalrRight2Dsply_B_Stat"
  BalrRight2Fast_B_Stat/1 -> bus_creator/4  "BalrRight2Fast_B_Stat"
  BalrRight2Prev1X_L_Actl/1 -> bus_creator/5  "BalrRight2Prev1X_L_Actl"
  BalrRight2Prev1Y_L_Actl/1 -> bus_creator/6  "BalrRight2Prev1Y_L_Actl"
  BalrRight2Prev2X_L_Actl/1 -> bus_creator/7  "BalrRight2Prev2X_L_Actl"
  BalrRight2Prev2Y_L_Actl/1 -> bus_creator/8  "BalrRight2Prev2Y_L_Actl"
  BalrRight2Prev3X_L_Actl/1 -> bus_creator/9  "BalrRight2Prev3X_L_Actl"
  BalrRight2Prev3Y_L_Actl/1 -> bus_creator/10  "BalrRight2Prev3Y_L_Actl"
  BalrRight2Threat_D_Stat/1 -> bus_creator/11  "BalrRight2Threat_D_Stat"

== system test_mdl1/VehicleCAN/IPMA_ADAS/BoundaryAlert_Right_3 ==
  BalrRight3CurntX_L_Actl : Constant  Value=0
  BalrRight3CurntY_L_Actl : Constant  Value=0
  BalrRight3Dsply_B_Stat : Constant  Value=0
  BalrRight3Fast_B_Stat : Constant  Value=0
  BalrRight3Prev1X_L_Actl : Constant  Value=0
  BalrRight3Prev1Y_L_Actl : Constant  Value=0
  BalrRight3Prev2X_L_Actl : Constant  Value=0
  BalrRight3Prev2Y_L_Actl : Constant  Value=0
  BalrRight3Prev3X_L_Actl : Constant  Value=0
  BalrRight3Prev3Y_L_Actl : Constant  Value=0
  BalrRight3Threat_D_Stat : Constant  Value=0
  bus_creator : BusCreator  Inputs=11
  out_port : Outport
  wires:
  bus_creator/1 -> out_port/1  "test_mdl1"
  BalrRight3CurntX_L_Actl/1 -> bus_creator/1  "BalrRight3CurntX_L_Actl"
  BalrRight3CurntY_L_Actl/1 -> bus_creator/2  "BalrRight3CurntY_L_Actl"
  BalrRight3Dsply_B_Stat/1 -> bus_creator/3  "BalrRight3Dsply_B_Stat"
  BalrRight3Fast_B_Stat/1 -> bus_creator/4  "BalrRight3Fast_B_Stat"
  BalrRight3Prev1X_L_Actl/1 -> bus_creator/5  "BalrRight3Prev1X_L_Actl"
  BalrRight3Prev1Y_L_Actl/1 -> bus_creator/6  "BalrRight3Prev1Y_L_Actl"
  BalrRight3Prev2X_L_Actl/1 -> bus_creator/7  "BalrRight3Prev2X_L_Actl"
  BalrRight3Prev2Y_L_Actl/1 -> bus_creator/8  "BalrRight3Prev2Y_L_Actl"
  BalrRight3Prev3X_L_Actl/1 -> bus_creator/9  "BalrRight3Prev3X_L_Actl"
  BalrRight3Prev3Y_L_Actl/1 -> bus_creator/10  "BalrRight3Prev3Y_L_Actl"
  BalrRight3Threat_D_Stat/1 -> bus_creator/11  "BalrRight3Threat_D_Stat"

== system test_mdl1/VehicleCAN/IPMA_ADAS/BoundaryAlert_Right_4 ==
  BalrRight4CurntX_L_Actl : Constant  Value=0
  BalrRight4CurntY_L_Actl : Constant  Value=0
  BalrRight4Dsply_B_Stat : Constant  Value=0
  BalrRight4Fast_B_Stat : Constant  Value=0
  BalrRight4Prev1X_L_Actl : Constant  Value=0
  BalrRight4Prev1Y_L_Actl : Constant  Value=0
  BalrRight4Prev2X_L_Actl : Constant  Value=0
  BalrRight4Prev2Y_L_Actl : Constant  Value=0
  BalrRight4Prev3X_L_Actl : Constant  Value=0
  BalrRight4Prev3Y_L_Actl : Constant  Value=0
  BalrRight4Threat_D_Stat : Constant  Value=0
  bus_creator : BusCreator  Inputs=11
  out_port : Outport
  wires:
  bus_creator/1 -> out_port/1  "test_mdl1"
  BalrRight4CurntX_L_Actl/1 -> bus_creator/1  "BalrRight4CurntX_L_Actl"
  BalrRight4CurntY_L_Actl/1 -> bus_creator/2  "BalrRight4CurntY_L_Actl"
  BalrRight4Dsply_B_Stat/1 -> bus_creator/3  "BalrRight4Dsply_B_Stat"
  BalrRight4Fast_B_Stat/1 -> bus_creator/4  "BalrRight4Fast_B_Stat"
  BalrRight4Prev1X_L_Actl/1 -> bus_creator/5  "BalrRight4Prev1X_L_Actl"
  BalrRight4Prev1Y_L_Actl/1 -> bus_creator/6  "BalrRight4Prev1Y_L_Actl"
  BalrRight4Prev2X_L_Actl/1 -> bus_creator/7  "BalrRight4Prev2X_L_Actl"
  BalrRight4Prev2Y_L_Actl/1 -> bus_creator/8  "BalrRight4Prev2Y_L_Actl"
  BalrRight4Prev3X_L_Actl/1 -> bus_creator/9  "BalrRight4Prev3X_L_Actl"
  BalrRight4Prev3Y_L_Actl/1 -> bus_creator/10  "BalrRight4Prev3Y_L_Actl"
  BalrRight4Threat_D_Stat/1 -> bus_creator/11  "BalrRight4Threat_D_Stat"

== system test_mdl1/VehicleCAN/IPMA_ADAS/GlareFreeBeam ==
  AdbBeam_D_Rq : Constant  Value=0
  AdbBrdrBottom_An_Rq : Constant  Value=0
  AdbBrdrLeft_An_Rq : Constant  Value=0
  AdbBrdrLeft_L_Stat : Constant  Value=0
  AdbBrdrRight_An_Rq : Constant  Value=0
  AdbBrdrRight_L_Stat : Constant  Value=0
  AdbBrdrTop_An_Rq : Constant  Value=0
  AdbRamping_T_Rq : Constant  Value=0
  bus_creator : BusCreator  Inputs=8
  out_port : Outport
  wires:
  bus_creator/1 -> out_port/1  "test_mdl1"
  AdbBeam_D_Rq/1 -> bus_creator/1  "AdbBeam_D_Rq"
  AdbBrdrBottom_An_Rq/1 -> bus_creator/2  "AdbBrdrBottom_An_Rq"
  AdbBrdrLeft_An_Rq/1 -> bus_creator/3  "AdbBrdrLeft_An_Rq"
  AdbBrdrLeft_L_Stat/1 -> bus_creator/4  "AdbBrdrLeft_L_Stat"
  AdbBrdrRight_An_Rq/1 -> bus_creator/5  "AdbBrdrRight_An_Rq"
  AdbBrdrRight_L_Stat/1 -> bus_creator/6  "AdbBrdrRight_L_Stat"
  AdbBrdrTop_An_Rq/1 -> bus_creator/7  "AdbBrdrTop_An_Rq"
  AdbRamping_T_Rq/1 -> bus_creator/8  "AdbRamping_T_Rq"

== system test_mdl1/VehicleCAN/IPMA_ADAS/IPMA_Data ==
  %sIndexIpma_D_Actl : Constant  Value=0
  AhbHiBeam_D_Rq : Constant  Value=0
  AhbcRampingV_D_Rq : Constant  Value=0
  CamraDefog_B_Req : Constant  Value=0
  CamraStats_D_Dsply : Constant  Value=0
  DasAlrtLvl_D_Dsply : Constant  Value=0
  DasStats_D_Dsply : Constant  Value=0
  DasWarn_D_Dsply : Constant  Value=0
  FeatConfigIpmaActl : Constant  Value=0
  FeatNoIpmaActl : Constant  Value=0
  LaActvStats_D_Dsply : Constant  Value=0
  LaDenyStats_B_Dsply : Constant  Value=0
  LaHandsOff_D_Dsply : Constant  Value=0
  bus_creator : BusCreator  Inputs=13
  out_port : Outport
  wires:
  bus_creator/1 -> out_port/1  "test_mdl1"
  AhbHiBeam_D_Rq/1 -> bus_creator/1  "AhbHiBeam_D_Rq"
  AhbcRampingV_D_Rq/1 -> bus_creator/2  "AhbcRampingV_D_Rq"
  CamraDefog_B_Req/1 -> bus_creator/3  "CamraDefog_B_Req"
  CamraStats_D_Dsply/1 -> bus_creator/4  "CamraStats_D_Dsply"
  DasAlrtLvl_D_Dsply/1 -> bus_creator/5  "DasAlrtLvl_D_Dsply"
  DasStats_D_Dsply/1 -> bus_creator/6  "DasStats_D_Dsply"
  DasWarn_D_Dsply/1 -> bus_creator/7  "DasWarn_D_Dsply"
  FeatConfigIpmaActl/1 -> bus_creator/8  "FeatConfigIpmaActl"
  FeatNoIpmaActl/1 -> bus_creator/9  "FeatNoIpmaActl"
  LaActvStats_D_Dsply/1 -> bus_creator/10  "LaActvStats_D_Dsply"
  LaDenyStats_B_Dsply/1 -> bus_creator/11  "LaDenyStats_B_Dsply"
  LaHandsOff_D_Dsply/1 -> bus_creator/12  "LaHandsOff_D_Dsply"
  %sIndexIpma_D_Actl/1 -> bus_creator/13  "%sIndexIpma_D_Actl"

== system test_mdl1/VehicleCAN/IPMA_ADAS/IPMA_Data2 ==
  AdbDividedRoad_B_Stat : Constant  Value=0
  AdbDrvSide_B_Stat : Constant  Value=0
  DasAlrtInfo_D_Dsply : Constant  Value=0
  IaccVLimUnit_D_Rq : Constant  Value=0
  IaccVLim_D_Rq : Constant  Value=0
  IsaVLimUnit_D_Rq : Constant  Value=0
  IsaVLim_D_Rq : Constant  Value=0
  LcwaMsgTxt_D_Stat : Constant  Value=0
  LdwChime_B_Rq : Constant  Value=0
  LongCtrlEnbl_D_Rq : Constant  Value=0
  SblmPedCrossScnr_B_Stat : Constant  Value=0
  SblmRndAbtScnr_B_Stat : Constant  Value=0
  SblmStopScnr_B_Stat : Constant  Value=0
  SblmYieldScnr_B_Stat : Constant  Value=0
  TsrRegionTxt_D_Stat : Constant  Value=0
  bus_creator : BusCreator  Inputs=15
  out_port : Outport
  wires:
  bus_creator/1 -> out_port/1  "test_mdl1"
  AdbDividedRoad_B_Stat/1 -> bus_creator/1  "AdbDividedRoad_B_Stat"
  AdbDrvSide_B_Stat/1 -> bus_creator/2  "AdbDrvSide_B_Stat"
  DasAlrtInfo_D_Dsply/1 -> bus_creator/3  "DasAlrtInfo_D_Dsply"
  IaccVLimUnit_D_Rq/1 -> bus_creator/4  "IaccVLimUnit_D_Rq"
  IaccVLim_D_Rq/1 -> bus_creator/5  "IaccVLim_D_Rq"
  IsaVLimUnit_D_Rq/1 -> bus_creator/6  "IsaVLimUnit_D_Rq"
  IsaVLim_D_Rq/1 -> bus_creator/7  "IsaVLim_D_Rq"
  LcwaMsgTxt_D_Stat/1 -> bus_creator/8  "LcwaMsgTxt_D_Stat"
  LdwChime_B_Rq/1 -> bus_creator/9  "LdwChime_B_Rq"
  LongCtrlEnbl_D_Rq/1 -> bus_creator/10  "LongCtrlEnbl_D_Rq"
  SblmPedCrossScnr_B_Stat/1 -> bus_creator/11  "SblmPedCrossScnr_B_Stat"
  SblmRndAbtScnr_B_Stat/1 -> bus_creator/12  "SblmRndAbtScnr_B_Stat"
  SblmStopScnr_B_Stat/1 -> bus_creator/13  "SblmStopScnr_B_Stat"
  SblmYieldScnr_B_Stat/1 -> bus_creator/14  "SblmYieldScnr_B_Stat"
  TsrRegionTxt_D_Stat/1 -> bus_creator/15  "TsrRegionTxt_D_Stat"
